simulink model "model"  (R2025b)
settings: Solver=VariableStepAuto  StartTime=0.0  StopTime=10000  RelTol=1e-3
values from neighbouring files (symbols this model uses):
  A = double(subs(Aj, [h1_tmp, h2_tmp, Qin_tmp], [h_calced, h_calced, Qin]))    [script.m]
  A_inv = 1/ A    (= 0.25)    [script.m]
  B = double(subs(Bj, [h1_tmp, h2_tmp, Qin_tmp], [h_calced, h_calced, Qin]))    [script.m]
  C = [1, 0 ... (first row only)    [script.m]
  D = [0 ... (first row only)    [script.m]
  h_calced = (Qin / S)^2 / (2 * g)    (= 0.815494393476)    [script.m]
  k_valve = S * sqrt(2 * g)    [script.m]
  Qin = 10 / 1000    (= 0.01)    [script.m]
  Qin_step = 30    [script.m]
  T_step = 10000    [script.m]
undefined symbols (not defined in the file or in its folder): den1, den2, num1, num2
settings Model: Creator=Vladimir  LastModifiedBy=Vladimir

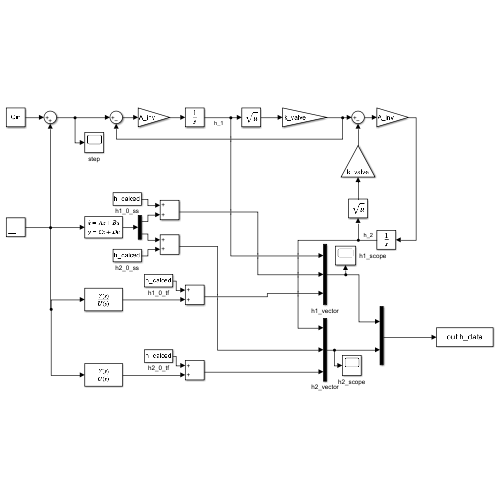
[thumbnail: Simulink's stored preview of the top-level diagram]
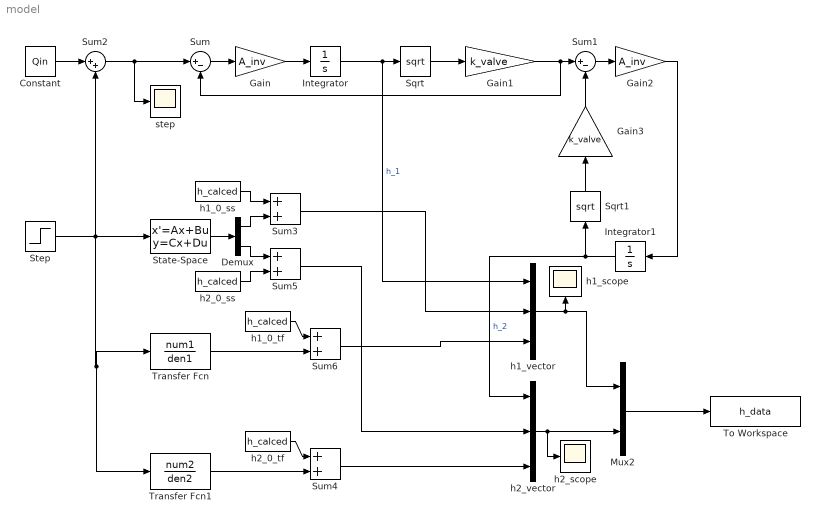
== system model ==
  Constant : Constant  Value=Qin
  Demux : Demux  Outputs=2
  Gain : Gain  Gain=A_inv
  Gain1 : Gain  Gain=k_valve
  Gain2 : Gain  Gain=A_inv
  Gain3 : Gain  Gain=k_valve
  Integrator : Integrator  InitialCondition=h_calced
  Integrator1 : Integrator  InitialCondition=h_calced
  Mux2 : Mux  Inputs=2
  Sqrt : Sqrt
  Sqrt1 : Sqrt
  State-Space : StateSpace  A=A  B=B  C=C  D=D  InitialCondition=0
  Step : Step  Time=T_step  After=Qin_step / 10000  SampleTime=0
  Sum : Sum  Inputs=|+-
  Sum1 : Sum  Inputs=|+-
  Sum2 : Sum  Inputs=|++
  Sum{3..6} (4 alike) : Sum
  To Workspace : ToWorkspace  VariableName=h_data  SaveFormat=Timeseries  SampleTime=-1
  Transfer Fcn : TransferFcn  Numerator=num1  Denominator=den1
  Transfer Fcn1 : TransferFcn  Numerator=num2  Denominator=den2
  h1_0_ss : Constant  Value=h_calced
  h1_0_tf : Constant  Value=h_calced
  h1_scope : Scope
      settings: ActiveDisplayYMinimum=-1  ActiveDisplayYMaximum=1
  h1_vector : Mux  Inputs=3
  h2_0_ss : Constant  Value=h_calced
  h2_0_tf : Constant  Value=h_calced
  h2_scope : Scope
      settings: ActiveDisplayYMinimum=-1  ActiveDisplayYMaximum=1  DataLoggingVariableName=ScopeData2
  h2_vector : Mux  Inputs=3
  step : Scope
      settings: ActiveDisplayYMinimum=-1  ActiveDisplayYMaximum=1
  wires:
  Constant/1 -> Sum2/1
  Sum/1 -> Gain/1
  Gain/1 -> Integrator/1
  Integrator/1 -> h1_vector/1, Sqrt/1  "h_1"
  Sqrt/1 -> Gain1/1
  Gain1/1 -> Sum/2, Sum1/1
  Sum1/1 -> Gain2/1
  Gain2/1 -> Integrator1/1
  Integrator1/1 -> Sqrt1/1, h2_vector/1  "h_2"
  Sqrt1/1 -> Gain3/1
  Gain3/1 -> Sum1/2
  Step/1 -> Sum2/2, Transfer Fcn1/1, Transfer Fcn/1, State-Space/1
  Sum2/1 -> step/1, Sum/1
  State-Space/1 -> Demux/1
  Demux/1 -> Sum3/2
  Demux/2 -> Sum5/1
  h1_0_ss/1 -> Sum3/1
  h2_0_tf/1 -> Sum4/1
  h1_0_tf/1 -> Sum6/1
  Transfer Fcn/1 -> Sum6/2
  Transfer Fcn1/1 -> Sum4/2
  h2_0_ss/1 -> Sum5/2
  Sum5/1 -> h2_vector/2
  Sum4/1 -> h2_vector/3
  Sum3/1 -> h1_vector/2
  Sum6/1 -> h1_vector/3
  h1_vector/1 -> h1_scope/1, Mux2/1
  h2_vector/1 -> Mux2/2, h2_scope/1
  Mux2/1 -> To Workspace/1
